simulink model "s0509_rollest_rideheight_noaxleroll"  (R2021a)
settings: Solver=FixedStepAuto  StartTime=0.0  StopTime=10.0  FixedStep=0.001  RelTol=1e-3
undefined symbols (not defined in the file or in its folder): Ts, Tsample2ms
libraries: CarMaker4SL x36, dspfdesign x1, simulink x1
settings Model: Creator=jason  LastModifiedBy=jason
settings ModelReferenceCC: ModelReferenceNumInstancesAllowed=Single

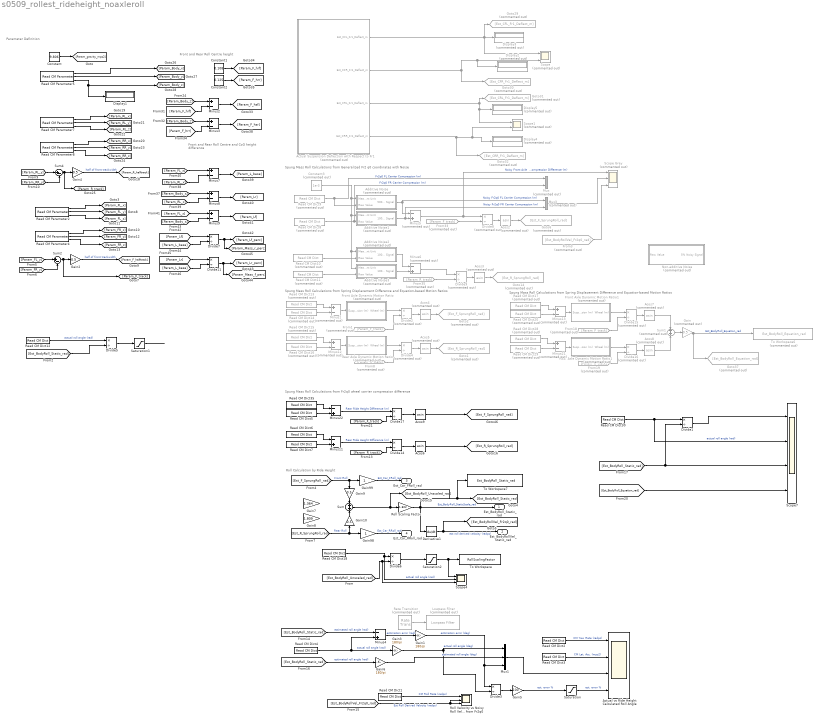
== system s0509_rollest_rideheight_noaxleroll ==
  note: Front and Rear Roll Centre height
  note: Roll Calculation by Ride Height
  note: Parameter Definition
  note: Spung Mass Roll Calculations from Generalized Fr2 q0 coordinates with Noise
  note: Front and Rear Roll Centre and CoG height difference
  note: Spung Mass Roll Calculations from Spring Displacement Difference and Equation-based Motion Ratios
  note: Spung Mass Roll Calculations from Fr2q0 wheel carrier compression difference
  note: Spung Mass Roll Calculations from Spring Displacement Difference and Equation-based Motion Ratios
  Acos{2..5,7..8} (6 alike) : Trigonometry  Commented=on  Operator=asin
  Acos6 : Trigonometry  Operator=asin
  Acos9 : Trigonometry  Operator=asin
  Actual Suspension Deflection with Respect to Fr1 : Subsystem  Commented=on
  Actual vs Ride Height Calculated Roll Angle : Scope  NumInputPorts=4
  Additive Noise : Subsystem  Commented=on
  Additive Noise1 : Subsystem  Commented=on
  Additive Noise2 : Subsystem  Commented=on
  Additive Noise3 : Subsystem  Commented=on
  Constant : Constant  Value=9.806
  Constant1 : Constant  Value=0.108
  Constant2 : Constant  Value=0.125
  Constant3 : Constant  Commented=on  Value=1e-3
  Derivative1 : Derivative
  Display1 : Display
  Display{2..5} (4 alike) : Display  Commented=on
  Divide{1,3,5..7,11,14,17} (8 alike) : Product  Inputs=*/
  Divide{2,4,8..9,15..16} (6 alike) : Product  Commented=on  Inputs=*/
  From1 : From  Commented=on  GotoTag=Param_F_track
  From18 : From  Commented=on  GotoTag=Param_F_track
  From19 : From  Commented=on  GotoTag=Param_R_track
  From3 : From  Commented=on  GotoTag=Est_BodyRollVel_Fr2q0_rad
  From33 : From  Commented=on  GotoTag=Param_F_track
  From35 : From  Commented=on  GotoTag=Param_R_track
  From8 : From  Commented=on  GotoTag=Param_R_track
  Front Axle Dynamic Motion Ratio : Subsystem  Commented=on
  Front Axle Dynamic Motion Ratio1 : Subsystem  Commented=on
  Gain : Gain  Commented=on  Gain=0.5
  Gain1 : Gain  Gain=180/pi
      settings: AttributesFormatString=Gain = %<Gain>
  Gain{2,4,9..10} (4 alike) : Gain  Gain=0.5
  Gain3 : Gain  Gain=180/pi
      settings: AttributesFormatString=Gain = %<Gain>
  Gain5 : Gain  Gain=100
  Gain6 : Gain  Gain=180/pi
      settings: AttributesFormatString=Gain = %<Gain>
  Gain7 : Gain  Gain=1.364
  Gain8 : Gain  Gain=1.809
  Gain98 : Gain
  Gain99 : Gain
  Goto1 : Goto  Commented=on  GotoTag=Est_R_SprungRoll_rad
  Goto14 : Goto  Commented=on  GotoTag=Est_R_SprungRoll_rad
  Goto2 : Goto  Commented=on  GotoTag=Est_F_SprungRoll_rad
  Goto29 : Goto  Commented=on  GotoTag=Est_CFL_Fr1_Deflect_m
  Goto30 : Goto  Commented=on  GotoTag=Est_CFR_Fr1_Deflect_m
  Goto31 : Goto  Commented=on  GotoTag=Est_CRL_Fr1_Deflect_m
  Goto32 : Goto  Commented=on  GotoTag=Est_CRR_Fr1_Deflect_m
  Goto37 : Goto  Commented=on  GotoTag=Est_BodyRoll_Equation_rad
  Goto6 : Goto  Commented=on  GotoTag=Est_F_SprungRoll_rad
  Lowpass Filter : dspfdesign/Lowpass Filter  Commented=on  FilterType=FIR  DesignForMinimumOrder=on  FilterOrder=50  PassbandFrequency=1  StopbandFrequency=2000  PassbandRipple=0.1  StopbandAttenuation=180  InheritSampleRate=off  SampleRate=44100  SimulateUsing=Interpreted execution  roundingMode=Floor  coeffsDataTypeStr=fixdt(1,16)
  Minus{1,12..13,21} (4 alike) : Sum  Commented=on  Inputs=+-
  Minus11 : Sum  Inputs=-+
  Minus{2..3,7..9} (5 alike) : Sum  Inputs=+-
  Minus22 : Sum  Inputs=-+
  Minus4 : Sum  Inputs=-+
  Minus5 : Sum  Commented=on  Inputs=-+
  Minus6 : Sum  Commented=on  Inputs=-+
  Mux : Mux  Commented=on  Inputs=2
  Mux1 : Mux  Inputs=3
  Mux3 : Mux  Commented=on  Inputs=2
  Non-additive Noise : Subsystem  Commented=on
  Rate Transition : RateTransition  Commented=on
  Read CM Dict1 : CarMaker4SL/Read CM Dict  xname=Car.RollVel  xsync=off  xstime=Continuous
  Read CM Dict10 : CarMaker4SL/Read CM Dict  Commented=on  xname=Car.CRL.q0  xsync=off  xstime=Continuous
  Read CM Dict11 : CarMaker4SL/Read CM Dict  Commented=on  xname=Car.CRR.q0  xsync=off  xstime=Continuous
  Read CM Dict{4,12,18,30} (4 alike) : CarMaker4SL/Read CM Dict  xname=Car.Roll  xsync=off  xstime=Continuous
  Read CM Dict13 : CarMaker4SL/Read CM Dict  Commented=on  xname=Car.SpringFL.l  xsync=off  xstime=Continuous
  Read CM Dict14 : CarMaker4SL/Read CM Dict  Commented=on  xname=Car.SpringFR.l  xsync=off  xstime=Continuous
  Read CM Dict15 : CarMaker4SL/Read CM Dict  Commented=on  xname=Car.SpringRL.l  xsync=off  xstime=Continuous
  Read CM Dict16 : CarMaker4SL/Read CM Dict  Commented=on  xname=Car.SpringRR.l  xsync=off  xstime=Continuous
  Read CM Dict17 : CarMaker4SL/Read CM Dict  Commented=on  xname=Car.SpringFL.l  xsync=off  xstime=Continuous
  Read CM Dict2 : CarMaker4SL/Read CM Dict  xname=Car.YawRate  xsync=off  xstime=Continuous
  Read CM Dict20 : CarMaker4SL/Read CM Dict  Commented=on  xname=Car.SpringFR.l  xsync=off  xstime=Continuous
  Read CM Dict28 : CarMaker4SL/Read CM Dict  Commented=on  xname=Car.SpringRL.l  xsync=off  xstime=Continuous
  Read CM Dict29 : CarMaker4SL/Read CM Dict  Commented=on  xname=Car.SpringRR.l  xsync=off  xstime=Continuous
  Read CM Dict3 : CarMaker4SL/Read CM Dict  xname=Car.ay  xsync=off  xstime=Continuous
  Read CM Dict35 : CarMaker4SL/Read CM Dict  xname=Car.CFL.q0  xsync=off  xstime=Continuous
  Read CM Dict5 : CarMaker4SL/Read CM Dict  xname=Car.CFR.q0  xsync=off  xstime=Continuous
  Read CM Dict6 : CarMaker4SL/Read CM Dict  xname=Car.CRL.q0  xsync=off  xstime=Continuous
  Read CM Dict7 : CarMaker4SL/Read CM Dict  xname=Car.CRR.q0  xsync=off  xstime=Continuous
  Read CM Dict8 : CarMaker4SL/Read CM Dict  Commented=on  xname=Car.CFR.q0  xsync=off  xstime=Continuous
  Read CM Dict9 : CarMaker4SL/Read CM Dict  Commented=on  xname=Car.CFL.q0  xsync=off  xstime=Continuous
  Read CM Parameter2 : CarMaker4SL/Read CM Parameter  xfile=Vehicle  xkey=WheelCarrier.fl.pos  xnout=3  xdefaults=eps  xmuxed=off  xstime=Continuous
      settings: SourceProductName=CarMaker4SL
  Read CM Parameter4 : CarMaker4SL/Read CM Parameter  xfile=Vehicle  xkey=WheelCarrier.fr.pos  xnout=3  xdefaults=eps  xmuxed=off  xstime=Continuous
      settings: SourceProductName=CarMaker4SL
  Read CM Parameter5 : CarMaker4SL/Read CM Parameter  xfile=Vehicle  xkey=Body.pos  xnout=3  xdefaults=eps  xmuxed=off  xstime=Continuous
      settings: SourceProductName=CarMaker4SL
  Read CM Parameter7 : CarMaker4SL/Read CM Parameter  xfile=Vehicle  xkey=WheelCarrier.rl.pos  xnout=3  xdefaults=eps  xmuxed=off  xstime=Continuous
      settings: SourceProductName=CarMaker4SL
  Read CM Parameter8 : CarMaker4SL/Read CM Parameter  xfile=Vehicle  xkey=WheelCarrier.rr.pos  xnout=3  xdefaults=eps  xmuxed=off  xstime=Continuous
      settings: SourceProductName=CarMaker4SL
  Rear Axle Dynamic Motion Ratio : Subsystem  Commented=on
  Rear Axle Dynamic Motion Ratio1 : Subsystem  Commented=on
  Roll Scaling Factor : Gain  Gain=1.822
  Roll Velocity vs Noisy Roll Velocity from Fr2q0 : Scope  NumInputPorts=3
  Saturation : Saturate  UpperLimit=100  LowerLimit=-100
  Saturation1 : Saturate  UpperLimit=3.6  LowerLimit=1.25
  Saturation2 : Saturate  UpperLimit=3.6  LowerLimit=1.25
  Scope : Scope  Commented=on  NumInputPorts=3
  Scope Grey : Scope  Commented=on  NumInputPorts=3
  Scope1 : Scope  Commented=on  NumInputPorts=2
  Scope4 : Scope  NumInputPorts=3
  Scope7 : Scope  NumInputPorts=4
  Sum : Sum  Inputs=+|+
  Sum1 : Sum  Commented=on  Inputs=+|+
  Sum2 : Sum  Inputs=|+-
  Sum4 : Sum  Inputs=|+-
  To Workspace : ToWorkspace  VariableName=RollScalingFactor  SampleTime=-1
  To Workspace6 : ToWorkspace  Commented=on  VariableName=Est_BodyRoll_Equation_rad  SampleTime=-1
  To Workspace7 : ToWorkspace  VariableName=Est_BodyRoll_Static_rad  SampleTime=-1
  Est_BodyRoll_Static_rad : Outport
  Est_BodyRollVel_Static_rad : Outport  Port=2
  Est_Car_FRoll_rad : Outport  Port=3
  Est_Car_RRoll_rad : Outport  Port=4
  wires:
  From33/1 -> Divide8/2
  [Param_RR_y] -> Sum4/2
  Minus5/1 -> Scope Grey/1, Divide8/1  "Noisy Front Axle  Fr2q0 Carrier Compression Difference (m)"
  Acos2/1 -> Goto6/1
  Acos3/1 -> Goto14/1
  Read CM Parameter4/2 -> [Param_FR_y]
  Sum/1 -> Roll Scaling Factor/1, [Est_BodyRoll_Unscaled_rad]
  Divide9/1 -> Acos3/1
  Minus6/1 -> Divide9/1
  Actual Suspension Deflection with Respect to Fr1/1(Est_CFL_Fr1_Deflect_m) -> Goto29/1, Scope/1, Display3/1
  Divide8/1 -> Acos2/1
  Read CM Dict10/1 -> Additive Noise2/2(Raw Value)
  Read CM Dict9/1 -> Mux/1, Additive Noise/2(Raw Value)  "Fr2q0 FL Carrier Compression (m)"
  Read CM Dict8/1 -> Mux/2, Additive Noise1/2(Raw Value)  "Fr2q0 FR Carrier Compression (m)"
  Derivative1/1 -> [Est_BodyRollVel_Fr2q0_rad], Est_BodyRollVel_Static_rad/1  "est roll derived velocity (radps)"
  From35/1 -> Divide9/2
  Read CM Dict11/1 -> Additive Noise3/2(Raw Value)
  Read CM Parameter8/1 -> [Param_RR_x]
  Actual Suspension Deflection with Respect to Fr1/4(Est_CRR_Fr1_Deflect_m) -> Goto32/1, Display4/1, Scope1/2
  Read CM Parameter2/3 -> [Param_FL_z]
  Gain2/1 -> [Param_F_halftrack]  "half of front trackwidth"
  Read CM Parameter2/1 -> [Param_FL_x]
  [Est_F_SprungRoll_rad] -> Gain99/1, Gain9/1  "Front Roll"
  [Param_FL_y] -> Sum2/1
  Constant/1 -> [Param_gravity_mps2]
  Sum4/1 -> Gain4/1, [Param_R_track]
  Sum2/1 -> Gain2/1, [Param_F_track]
  Actual Suspension Deflection with Respect to Fr1/2(Est_CFR_Fr1_Deflect_m) -> Display2/1, Scope/3, Goto30/1
  Read CM Parameter5/2 -> [Param_Body_y]
  Read CM Parameter5/1 -> [Param_Body_x]
  [Param_RL_y] -> Sum4/1
  Read CM Parameter2/2 -> [Param_FL_y]
  Read CM Parameter5/3 -> Display1/1, [Param_Body_z]
  Gain4/1 -> [Param_R_halftrack]  "half of front trackwidth"
  [Param_FR_y] -> Sum2/2
  Read CM Parameter8/2 -> [Param_RR_y]
  Read CM Parameter4/3 -> [Param_FR_z]
  Read CM Parameter4/1 -> [Param_FR_x]
  Read CM Parameter7/1 -> [Param_RL_x]
  Actual Suspension Deflection with Respect to Fr1/3(Est_CRL_Fr1_Deflect_m) -> Goto31/1, Scope1/1, Display5/1
  Read CM Parameter8/3 -> [Param_RR_z]
  Read CM Parameter7/3 -> [Param_RL_z]
  Read CM Parameter7/2 -> [Param_RL_y]
  Constant1/1 -> [Param_F_hrf]
  Constant2/1 -> [Param_F_hrr]
  [Param_F_hrf] -> Minus2/2
  [Param_Body_z] -> Minus2/1
  Minus2/1 -> [Param_F_hsf]
  Minus3/1 -> [Param_F_hsr]
  [Param_Body_z] -> Minus3/1
  [Param_F_hrr] -> Minus3/2
  [Param_Body_x] -> Minus8/1
  [Param_RL_x] -> Minus7/2
  [Param_FL_x] -> Minus7/1
  Minus7/1 -> [Param_L_base]
  [Param_RL_x] -> Minus8/2
  Minus8/1 -> [Param_Lr]
  [Param_FL_x] -> Minus9/1
  [Param_Body_x] -> Minus9/2
  Minus9/1 -> [Param_Lf]
  [Param_Lf] -> Divide7/1
  [Param_L_base] -> Divide7/2
  Divide7/1 -> [Param_Mass_r_perc], [Param_Lf_perc]
  Divide11/1 -> [Param_Mass_f_perc], [Param_Lr_perc]
  [Param_L_base] -> Divide11/2
  [Param_Lr] -> Divide11/1
  Additive Noise/1(500% of Unit Noisy Signal) -> Mux3/1, Minus5/1  "Noisy Fr2q0 FL Carrier Compression (m)"
  Constant3/1 -> Additive Noise/1(Measurement Unit), Additive Noise1/1(Measurement Unit), Additive Noise3/1(Measurement Unit), Additive Noise2/1(Measurement Unit)
  Additive Noise1/1(100% of Unit Noisy Signal) -> Mux3/2, Minus5/2  "Noisy Fr2q0 FR Carrier Compression (m)"
  Additive Noise2/1(100% of Unit Noisy Signal) -> Minus6/1
  Additive Noise3/1(100% of Unit Noisy Signal) -> Minus6/2
  Acos5/1 -> Goto1/1
  Rear Axle Dynamic Motion Ratio/1(Wheel (m)) -> Divide4/1
  From1/1 -> Divide2/2
  Divide4/1 -> Acos5/1
  Acos4/1 -> Goto2/1
  From8/1 -> Divide4/2
  Divide2/1 -> Acos4/1
  [Est_R_SprungRoll_rad] -> Gain98/1, Gain10/1  "Rear Roll"
  Gain9/1 -> Sum/1
  Gain10/1 -> Sum/2
  Read CM Dict2/1 -> Actual vs Ride Height Calculated Roll Angle/1  "CM Yaw Rate (radps)"
  Gain6/1 -> Mux1/2  "estimated roll angle (deg)"
  Minus4/1 -> Gain1/1  "estimation error (rad)"
  Rate Transition/1 -> Lowpass Filter/1
  Saturation/1 -> Actual vs Ride Height Calculated Roll Angle/4  "est. error %"
  Gain3/1 -> Divide3/2, Mux1/1  "actual roll angle (deg)"
  Gain5/1 -> Saturation/1  "est. error %"
  Read CM Dict4/1 -> Minus4/2, Gain3/1  "actual roll angle (rad)"
  [Est_BodyRoll_Static_rad] -> Minus4/1  "estimated roll angle (rad)"
  [Est_BodyRoll_Static_rad] -> Gain6/1  "estimated roll angle (rad)"
  Divide3/1 -> Gain5/1
  Read CM Dict3/1 -> Actual vs Ride Height Calculated Roll Angle/2  "CM Lat. Acc. (mps2)"
  Gain1/1 -> Divide3/1, Mux1/3  "estimation error (deg)"
  Read CM Dict1/1 -> Roll Velocity vs Noisy Roll Velocity from Fr2q0/1  "CM Roll Rate (radps)"
  Mux1/1 -> Actual vs Ride Height Calculated Roll Angle/3
  [Est_BodyRollVel_Fr2q0_rad] -> Roll Velocity vs Noisy Roll Velocity from Fr2q0/2, Roll Velocity vs Noisy Roll Velocity from Fr2q0/3  "Est Roll Derived Velocity (radps)"
  Minus12/1 -> Rear Axle Dynamic Motion Ratio/1(Suspension (m))
  Read CM Dict16/1 -> Minus12/2
  Read CM Dict15/1 -> Minus12/1
  Read CM Dict14/1 -> Minus1/2
  Minus1/1 -> Front Axle Dynamic Motion Ratio/1(Suspension (m))
  Front Axle Dynamic Motion Ratio/1(Wheel (m)) -> Divide2/1
  Read CM Dict13/1 -> Minus1/1
  Read CM Dict7/1 -> Minus11/2
  Read CM Dict35/1 -> Minus22/1
  Read CM Dict6/1 -> Minus11/1
  Minus11/1 -> Divide14/1  "Rear Ride Height Difference (m)"
  [Param_R_track] -> Divide14/2
  Read CM Dict5/1 -> Minus22/2
  Divide14/1 -> Acos6/1
  Minus13/1 -> Front Axle Dynamic Motion Ratio1/1(Suspension (m))
  Front Axle Dynamic Motion Ratio1/1(Wheel (m)) -> Divide15/1
  Read CM Dict29/1 -> Minus21/2
  Read CM Dict17/1 -> Minus13/1
  Acos8/1 -> Sum1/2
  Acos7/1 -> Sum1/1
  Read CM Dict28/1 -> Minus21/1
  From18/1 -> Divide15/2
  Rear Axle Dynamic Motion Ratio1/1(Wheel (m)) -> Divide16/1
  Divide15/1 -> Acos7/1
  Minus21/1 -> Rear Axle Dynamic Motion Ratio1/1(Suspension (m))
  From19/1 -> Divide16/2
  Read CM Dict20/1 -> Minus13/2
  Divide16/1 -> Acos8/1
  Sum1/1 -> Gain/1
  Gain/1 -> Goto37/1, To Workspace6/1  "Est_BodyRoll_Equation_rad"
  [Est_BodyRoll_Static_rad] -> Divide1/2, Scope7/3
  [Est_BodyRoll_Equation_rad] -> Scope7/4
  Read CM Dict30/1 -> Scope7/2, Divide1/1  "actual roll angle (rad)"
  Acos6/1 -> [Est_R_SprungRoll_rad]
  [Param_F_track] -> Divide17/2
  Divide17/1 -> Acos9/1
  Minus22/1 -> Divide17/1  "Rear Ride Height Difference (m)"
  Divide1/1 -> Scope7/1
  Read CM Dict12/1 -> Divide5/1  "actual roll angle (rad)"
  [Est_BodyRoll_Static_rad] -> Divide5/2
  Divide5/1 -> Saturation1/1
  Saturation1/1 -> ?
  Acos9/1 -> [Est_F_SprungRoll_rad]
  Saturation2/1 -> Scope4/1, To Workspace/1
  Roll Scaling Factor/1 -> Derivative1/1, Est_BodyRoll_Static_rad/1, [Est_BodyRoll_Static_rad], To Workspace7/1  "Est_BodyRoll_StaticScale_rad"
  [Est_BodyRoll_Unscaled_rad] -> Scope4/3, Divide6/2
  Read CM Dict18/1 -> Scope4/2, Divide6/1  "actual roll angle (rad)"
  Divide6/1 -> Saturation2/1
  Gain99/1 -> Est_Car_FRoll_rad/1  "Est_Car_FRoll_rad"
  Gain98/1 -> Est_Car_RRoll_rad/1  "Est_Car_RRoll_rad"
  Mux3/1 -> Scope Grey/2
  From3/1 -> Scope Grey/3

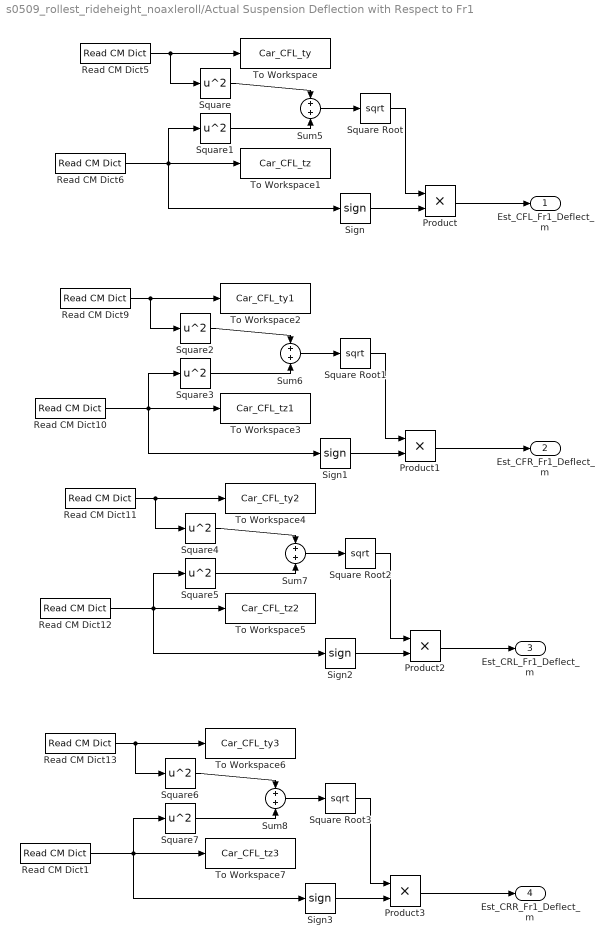
== system s0509_rollest_rideheight_noaxleroll/Actual Suspension Deflection with Respect to Fr1 ==
  Product{,1..3} (4 alike) : Product
  Read CM Dict1 : CarMaker4SL/Read CM Dict  xname=Car.CRR.tz  xsync=off  xstime=Continuous
  Read CM Dict10 : CarMaker4SL/Read CM Dict  xname=Car.CFR.tz  xsync=off  xstime=Continuous
  Read CM Dict11 : CarMaker4SL/Read CM Dict  xname=Car.CRL.ty  xsync=off  xstime=Continuous
  Read CM Dict12 : CarMaker4SL/Read CM Dict  xname=Car.CRL.tz  xsync=off  xstime=Continuous
  Read CM Dict13 : CarMaker4SL/Read CM Dict  xname=Car.CRR.ty  xsync=off  xstime=Continuous
  Read CM Dict5 : CarMaker4SL/Read CM Dict  xname=Car.CFL.ty  xsync=off  xstime=Continuous
  Read CM Dict6 : CarMaker4SL/Read CM Dict  xname=Car.CFL.tz  xsync=off  xstime=Continuous
  Read CM Dict9 : CarMaker4SL/Read CM Dict  xname=Car.CFR.ty  xsync=off  xstime=Continuous
  Sign{,1..3} (4 alike) : Signum
  Square{,1..7} (8 alike) : Math  Operator=square  SaturateOnIntegerOverflow=on
  Square Root{,1..3} (4 alike) : Sqrt  SaturateOnIntegerOverflow=on
  Sum{5..8} (4 alike) : Sum
  To Workspace : ToWorkspace  VariableName=Car_CFL_ty  SampleTime=-1
  To Workspace1 : ToWorkspace  VariableName=Car_CFL_tz  SampleTime=-1
  To Workspace2 : ToWorkspace  VariableName=Car_CFL_ty1  SampleTime=-1
  To Workspace3 : ToWorkspace  VariableName=Car_CFL_tz1  SampleTime=-1
  To Workspace4 : ToWorkspace  VariableName=Car_CFL_ty2  SampleTime=-1
  To Workspace5 : ToWorkspace  VariableName=Car_CFL_tz2  SampleTime=-1
  To Workspace6 : ToWorkspace  VariableName=Car_CFL_ty3  SampleTime=-1
  To Workspace7 : ToWorkspace  VariableName=Car_CFL_tz3  SampleTime=-1
  Est_CFL_Fr1_Deflect_m : Outport
  Est_CFR_Fr1_Deflect_m : Outport  Port=2
  Est_CRL_Fr1_Deflect_m : Outport  Port=3
  Est_CRR_Fr1_Deflect_m : Outport  Port=4
  wires:
  Square Root2/1 -> Product2/1
  Square Root1/1 -> Product1/1
  Read CM Dict11/1 -> Square4/1, To Workspace4/1
  Square Root/1 -> Product/1
  Sign2/1 -> Product2/2
  Square/1 -> Sum5/1
  Sum5/1 -> Square Root/1
  Sign/1 -> Product/2
  Square5/1 -> Sum7/2
  Sum7/1 -> Square Root2/1
  Read CM Dict12/1 -> Sign2/1, Square5/1, To Workspace5/1
  Read CM Dict10/1 -> Sign1/1, Square3/1, To Workspace3/1
  Square1/1 -> Sum5/2
  Read CM Dict5/1 -> Square/1, To Workspace/1
  Read CM Dict6/1 -> Sign/1, Square1/1, To Workspace1/1
  Read CM Dict9/1 -> Square2/1, To Workspace2/1
  Square3/1 -> Sum6/2
  Sum8/1 -> Square Root3/1
  Read CM Dict13/1 -> Square6/1, To Workspace6/1
  Square4/1 -> Sum7/1
  Square2/1 -> Sum6/1
  Square6/1 -> Sum8/1
  Sum6/1 -> Square Root1/1
  Read CM Dict1/1 -> Sign3/1, Square7/1, To Workspace7/1
  Square Root3/1 -> Product3/1
  Product1/1 -> Est_CFR_Fr1_Deflect_m/1
  Sign3/1 -> Product3/2
  Sign1/1 -> Product1/2
  Square7/1 -> Sum8/2
  Product2/1 -> Est_CRL_Fr1_Deflect_m/1
  Product/1 -> Est_CFL_Fr1_Deflect_m/1
  Product3/1 -> Est_CRR_Fr1_Deflect_m/1

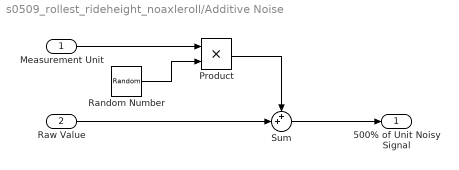
== system s0509_rollest_rideheight_noaxleroll/Additive Noise ==
  Measurement Unit : Inport
  Raw Value : Inport  Port=2
  Product : Product
  Random Number : RandomNumber  Variance=5  Seed=floor(rand(1)*25000)  SampleTime=Tsample2ms
  Sum : Sum  Inputs=++|
  500% of Unit Noisy Signal : Outport
  wires:
  Measurement Unit/1 -> Product/1
  Sum/1 -> 500% of Unit Noisy Signal/1
  Raw Value/1 -> Sum/2
  Product/1 -> Sum/1
  Random Number/1 -> Product/2

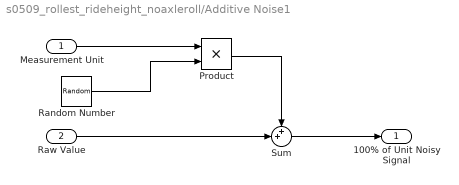
== system s0509_rollest_rideheight_noaxleroll/Additive Noise1 ==
  Measurement Unit : Inport
  Raw Value : Inport  Port=2
  Product : Product
  Random Number : RandomNumber  Variance=5  Seed=floor(rand(1)*25000)  SampleTime=Tsample2ms
  Sum : Sum  Inputs=++|
  100% of Unit Noisy Signal : Outport
  wires:
  Measurement Unit/1 -> Product/1
  Sum/1 -> 100% of Unit Noisy Signal/1
  Raw Value/1 -> Sum/2
  Product/1 -> Sum/1
  Random Number/1 -> Product/2

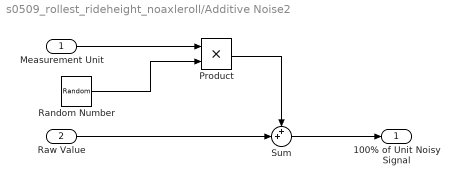
== system s0509_rollest_rideheight_noaxleroll/Additive Noise2 ==
  Measurement Unit : Inport
  Raw Value : Inport  Port=2
  Product : Product
  Random Number : RandomNumber  Variance=5  Seed=floor(rand(1)*25000)  SampleTime=Tsample2ms
  Sum : Sum  Inputs=++|
  100% of Unit Noisy Signal : Outport
  wires:
  Random Number/1 -> Product/2
  Product/1 -> Sum/1
  Raw Value/1 -> Sum/2
  Sum/1 -> 100% of Unit Noisy Signal/1
  Measurement Unit/1 -> Product/1

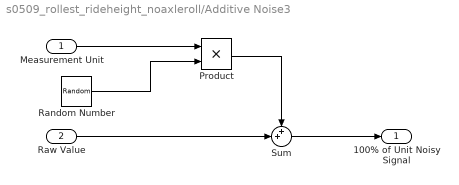
== system s0509_rollest_rideheight_noaxleroll/Additive Noise3 ==
  Measurement Unit : Inport
  Raw Value : Inport  Port=2
  Product : Product
  Random Number : RandomNumber  Variance=5  Seed=floor(rand(1)*25000)  SampleTime=Tsample2ms
  Sum : Sum  Inputs=++|
  100% of Unit Noisy Signal : Outport
  wires:
  Measurement Unit/1 -> Product/1
  Sum/1 -> 100% of Unit Noisy Signal/1
  Raw Value/1 -> Sum/2
  Product/1 -> Sum/1
  Random Number/1 -> Product/2

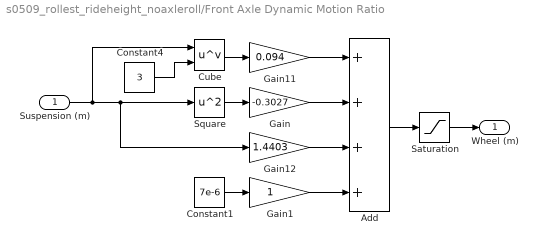
== system s0509_rollest_rideheight_noaxleroll/Front Axle Dynamic Motion Ratio ==
  Suspension (m) : Inport
  Add : Sum  Inputs=++++
  Constant1 : Constant  Value=7e-6
  Constant4 : Constant  Value=3
  Cube : Math  Operator=pow  SaturateOnIntegerOverflow=on
  Gain : Gain  Gain=-0.3027
  Gain1 : Gain
  Gain11 : Gain  Gain=0.094
  Gain12 : Gain  Gain=1.4403
  Saturation : Saturate  UpperLimit=1  LowerLimit=-1
  Square : Math  Operator=square  SaturateOnIntegerOverflow=on
  Wheel (m) : Outport
  wires:
  Suspension (m)/1 -> Cube/1, Gain12/1, Square/1
  Add/1 -> Saturation/1
  Cube/1 -> Gain11/1
  Gain/1 -> Add/2
  Gain12/1 -> Add/3
  Gain11/1 -> Add/1
  Square/1 -> Gain/1
  Constant1/1 -> Gain1/1
  Gain1/1 -> Add/4
  Constant4/1 -> Cube/2
  Saturation/1 -> Wheel (m)/1

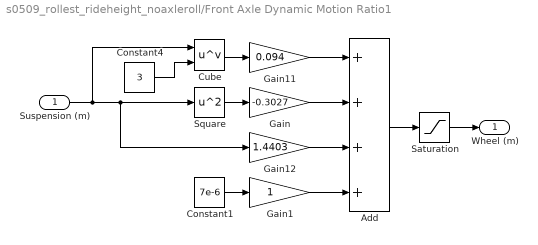
== system s0509_rollest_rideheight_noaxleroll/Front Axle Dynamic Motion Ratio1 ==
  Suspension (m) : Inport
  Add : Sum  Inputs=++++
  Constant1 : Constant  Value=7e-6
  Constant4 : Constant  Value=3
  Cube : Math  Operator=pow  SaturateOnIntegerOverflow=on
  Gain : Gain  Gain=-0.3027
  Gain1 : Gain
  Gain11 : Gain  Gain=0.094
  Gain12 : Gain  Gain=1.4403
  Saturation : Saturate  UpperLimit=1  LowerLimit=-1
  Square : Math  Operator=square  SaturateOnIntegerOverflow=on
  Wheel (m) : Outport
  wires:
  Suspension (m)/1 -> Cube/1, Gain12/1, Square/1
  Add/1 -> Saturation/1
  Cube/1 -> Gain11/1
  Gain/1 -> Add/2
  Gain12/1 -> Add/3
  Gain11/1 -> Add/1
  Square/1 -> Gain/1
  Constant1/1 -> Gain1/1
  Gain1/1 -> Add/4
  Constant4/1 -> Cube/2
  Saturation/1 -> Wheel (m)/1

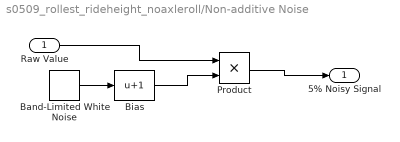
== system s0509_rollest_rideheight_noaxleroll/Non-additive Noise ==
  Raw Value : Inport
  Band-Limited White Noise : simulink/Sources/Band-Limited White Noise  Cov=[0.05]  Ts=Ts  seed=[23341]
  Bias : Bias  Bias=1
  Product : Product
  5% Noisy Signal : Outport
  wires:
  Band-Limited White Noise/1 -> Bias/1
  Bias/1 -> Product/2
  Raw Value/1 -> Product/1
  Product/1 -> 5% Noisy Signal/1

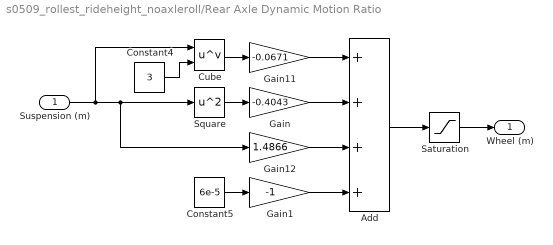
== system s0509_rollest_rideheight_noaxleroll/Rear Axle Dynamic Motion Ratio ==
  Suspension (m) : Inport
  Add : Sum  Inputs=++++
  Constant4 : Constant  Value=3
  Constant5 : Constant  Value=6e-5
  Cube : Math  Operator=pow  SaturateOnIntegerOverflow=on
  Gain : Gain  Gain=-0.4043
  Gain1 : Gain  Gain=-1
  Gain11 : Gain  Gain=-0.0671
  Gain12 : Gain  Gain=1.4866
  Saturation : Saturate  UpperLimit=1  LowerLimit=-1
  Square : Math  Operator=square  SaturateOnIntegerOverflow=on
  Wheel (m) : Outport
  wires:
  Square/1 -> Gain/1
  Gain11/1 -> Add/1
  Gain12/1 -> Add/3
  Constant4/1 -> Cube/2
  Gain/1 -> Add/2
  Cube/1 -> Gain11/1
  Add/1 -> Saturation/1
  Constant5/1 -> Gain1/1
  Suspension (m)/1 -> Cube/1, Square/1, Gain12/1
  Gain1/1 -> Add/4
  Saturation/1 -> Wheel (m)/1

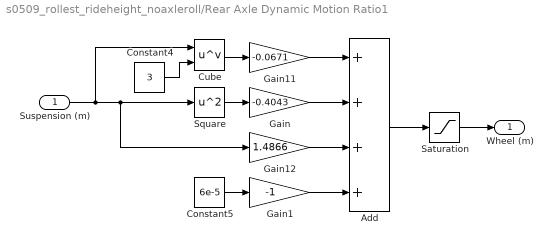
== system s0509_rollest_rideheight_noaxleroll/Rear Axle Dynamic Motion Ratio1 ==
  Suspension (m) : Inport
  Add : Sum  Inputs=++++
  Constant4 : Constant  Value=3
  Constant5 : Constant  Value=6e-5
  Cube : Math  Operator=pow  SaturateOnIntegerOverflow=on
  Gain : Gain  Gain=-0.4043
  Gain1 : Gain  Gain=-1
  Gain11 : Gain  Gain=-0.0671
  Gain12 : Gain  Gain=1.4866
  Saturation : Saturate  UpperLimit=1  LowerLimit=-1
  Square : Math  Operator=square  SaturateOnIntegerOverflow=on
  Wheel (m) : Outport
  wires:
  Square/1 -> Gain/1
  Gain11/1 -> Add/1
  Gain12/1 -> Add/3
  Constant4/1 -> Cube/2
  Gain/1 -> Add/2
  Cube/1 -> Gain11/1
  Add/1 -> Saturation/1
  Constant5/1 -> Gain1/1
  Suspension (m)/1 -> Cube/1, Square/1, Gain12/1
  Gain1/1 -> Add/4
  Saturation/1 -> Wheel (m)/1
